simulink model "Part2"  (R2024b)
settings: Solver=VariableStepAuto  StartTime=0.0  StopTime=10  RelTol=1e-3
InitFcn:
  | % Design2
values from neighbouring files (symbols this model uses):
  Ao = F(2, 2) - L * F(1, 2)    [Design1.m]    (also in Design2.m)
  Bo = [G(2) - L * G(1), Ao * L + F(2, 1) - L * F(1, 1)]    [Design1.m]    (also in Design2.m)
  Co = [0; 1]    [Design1.m]    (also in Design2.m)
  Do = [0, 1; 0, L]    [Design1.m]    (also in Design2.m)
  K = place(F, G, DesiredPoles)    [Design1.m]    (also in Design2.m = Ktmp(2:3))
  Nr = Nu + K * Nx    [Design1.m]    (also in Design2.m)
  Ts = TsCand(i)    [Design1.m]    (also in Design2.m)
undefined symbols (not defined in the file or in its folder): DiscIntNeverNeededParam, drv, F, G, H, J, sens
libraries: simulink_extras x5
settings Model: Creator=Banaan  LastModifiedBy=Banaan

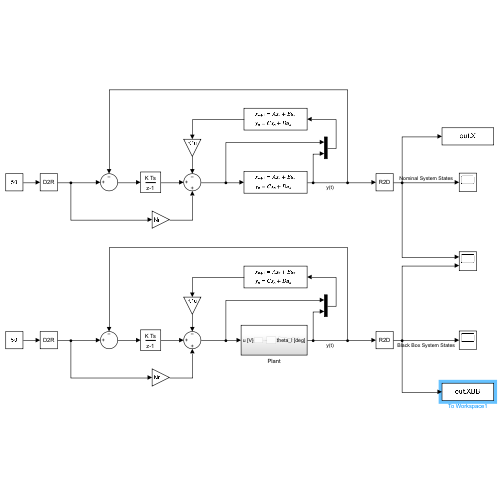
[thumbnail: Simulink's stored preview of the top-level diagram]
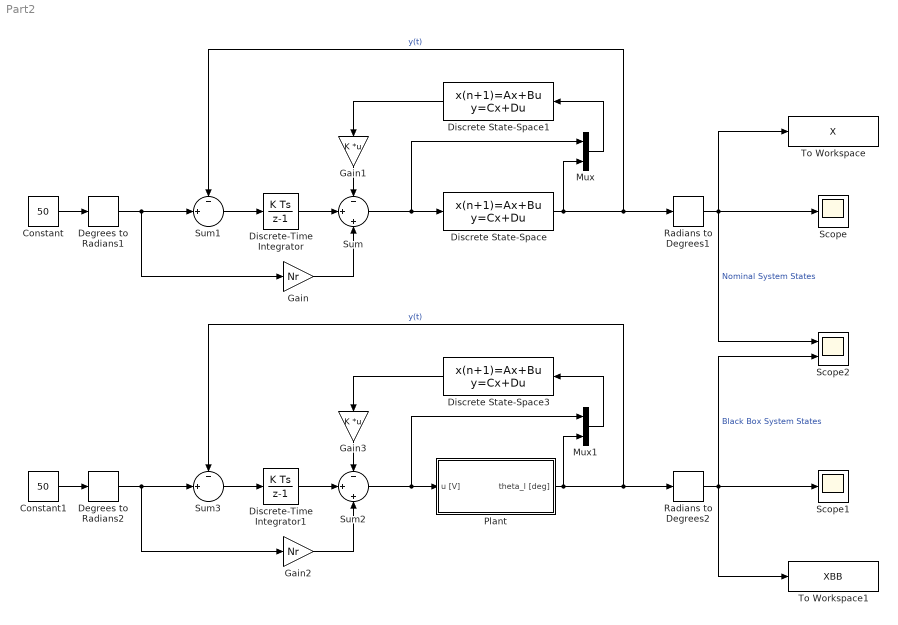
== system Part2 ==
  Constant : Constant  Value=50
  Constant1 : Constant  Value=50
  Degrees to Radians1 : simulink_extras/Transformations/Degrees to Radians
  Degrees to Radians2 : simulink_extras/Transformations/Degrees to Radians
  Discrete State-Space : DiscreteStateSpace  A=F  B=G  C=H  D=J  SampleTime=Ts
  Discrete State-Space1 : DiscreteStateSpace  A=Ao  B=Bo  C=Co  D=Do  SampleTime=Ts
  Discrete State-Space3 : DiscreteStateSpace  A=Ao  B=Bo  C=Co  D=Do  SampleTime=Ts
  Discrete-Time Integrator : DiscreteIntegrator  gainval=Ki  SampleTime=-1  ICPrevOutput=DiscIntNeverNeededParam  ICPrevScaledInput=DiscIntNeverNeededParam
  Discrete-Time Integrator1 : DiscreteIntegrator  gainval=Ki  SampleTime=-1  ICPrevOutput=DiscIntNeverNeededParam  ICPrevScaledInput=DiscIntNeverNeededParam
  Gain : Gain  Gain=Nr
  Gain1 : Gain  Gain=K  Multiplication=Matrix(K*u)
  Gain2 : Gain  Gain=Nr
  Gain3 : Gain  Gain=K  Multiplication=Matrix(K*u)
  Mux : Mux  Inputs=2
  Mux1 : Mux  Inputs=2
  Plant : Subsystem
  Radians to Degrees1 : simulink_extras/Transformations/Radians to Degrees
  Radians to Degrees2 : simulink_extras/Transformations/Radians to Degrees
  Scope : Scope
  Scope1 : Scope
  Scope2 : Scope  NumInputPorts=2
  Sum : Sum  Inputs=-|+|+
  Sum1 : Sum  Inputs=-|+||
  Sum2 : Sum  Inputs=-|+|+
  Sum3 : Sum  Inputs=-|+||
  To Workspace : ToWorkspace  VariableName=X  SaveFormat=Timeseries  SampleTime=-1
  To Workspace1 : ToWorkspace  VariableName=XBB  SaveFormat=Timeseries  SampleTime=-1
  wires:
  Constant/1 -> Degrees to Radians1/1
  Discrete State-Space/1 -> Mux/2, Radians to Degrees1/1, Sum1/1  "y(t)"
  Mux/1 -> Discrete State-Space1/1
  Sum/1 -> Mux/1, Discrete State-Space/1
  Discrete State-Space1/1 -> Gain1/1
  Gain/1 -> Sum/3
  Gain1/1 -> Sum/1
  Degrees to Radians1/1 -> Gain/1, Sum1/2
  Radians to Degrees1/1 -> To Workspace/1, Scope2/1, Scope/1  "Nominal System States"
  Discrete-Time Integrator/1 -> Sum/2
  Sum1/1 -> Discrete-Time Integrator/1
  Sum3/1 -> Discrete-Time Integrator1/1
  Discrete-Time Integrator1/1 -> Sum2/2
  Radians to Degrees2/1 -> To Workspace1/1, Scope2/2, Scope1/1  "Black Box System States"
  Degrees to Radians2/1 -> Sum3/2, Gain2/1
  Gain3/1 -> Sum2/1
  Gain2/1 -> Sum2/3
  Discrete State-Space3/1 -> Gain3/1
  Sum2/1 -> Plant/1(u [V]), Mux1/1
  Mux1/1 -> Discrete State-Space3/1
  Plant/1(theta_l [deg]) -> Sum3/1, Radians to Degrees2/1, Mux1/2  "y(t)"
  Constant1/1 -> Degrees to Radians2/1

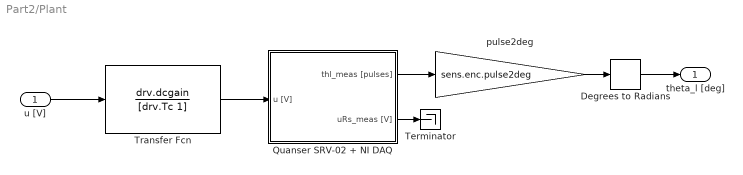
== system Part2/Plant ==
  u [V] : Inport
  Degrees to Radians : simulink_extras/Transformations/Degrees to Radians
  Quanser SRV-02 + NI DAQ : Subsystem  mask(Quanser SRV-02 (with inertial load) + NI DAQ){Ts=0.001, fricType=Coulomb + viscous}
      mask prompts: Ts "NI DAQ Sample Time:"; fricType "Friction model"
      mask help: Quanser SRV-02 (with inertial load) + NI DAQ model.
      mask init:
      | %%  Sensors data
      | 
      | %   shunt resistor
      | sens.curr.Rs = 0.5;                         %   resistance [Ohm]   
      | sens.curr.uRs_std = 0.01;                   %   voltage noise standard dev [V]                           
      | sens.curr.uRs_var = sens.curr.uRs_std^2;	%   voltage noise variance [V^2]
      | 
      | %   Hewlett-Packard HEDS-5540#A06 optical encoder
      | sens.enc.ppr = 500*4;                       %   pulses per rotation
      | sens.enc.pulse2deg = 360/sens.enc.ppr;      %   [pulses] -> [deg]
      | sens.enc.pulse2rad = 2*pi/sens.enc.ppr;     %   [pulses] -> [rad]
      | sens.enc.deg2pulse = sens.enc.ppr/360;      %   [deg] -> [pulses]
      | sens.enc.rad2pulse = sens.enc.ppr/2/pi;     %   [rad] -> [pulses]
      | 
      | 
      | %%  Data acquisition board (daq) data
      | 
      | %   NI PCI-6221 DAC data
      | daq.dac.bits = 16;                                  %   resolution (bits)
      | daq.dac.fs   = 10;                                  %   full scale 
      | daq.dac.q    = 2*daq.dac.fs/(2^daq.dac.bits-1);     %	quantization
      | 
      | %   NI PCI-6221 ADC data
      | daq.adc.bits = 16;                                  %   resolution (bits)
      | daq.adc.fs   = 10;                                  %   full scale (as set in SLDRT Analog Input block)
      | daq.adc.q    = 2*daq.adc.fs/(2^daq.adc.bits-1);     %   quantization
      mask Help:
      | Riccardo Antonello (antonello@dei.unipd.it)
      | 
      | April 24, 2020
      | 
      | Dept. of Information Engineering, University of Padova
      mask TypeOptions fricType: Coulomb + viscous | Karnopp
  Terminator : Terminator
  Transfer Fcn : TransferFcn  Numerator=drv.dcgain  Denominator=[drv.Tc 1]
  pulse2deg : Gain  Gain=sens.enc.pulse2deg
  theta_l [deg] : Outport
  wires:
  u [V]/1 -> Transfer Fcn/1
  Degrees to Radians/1 -> theta_l [deg]/1
  Quanser SRV-02 + NI DAQ/1(thl_meas [pulses]) -> pulse2deg/1
  Quanser SRV-02 + NI DAQ/2(uRs_meas [V]) -> Terminator/1
  Transfer Fcn/1 -> Quanser SRV-02 + NI DAQ/1(u [V])
  pulse2deg/1 -> Degrees to Radians/1

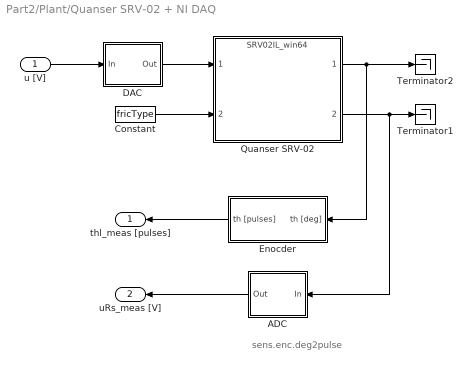
== system Part2/Plant/Quanser SRV-02 + NI DAQ ==
  note: sens.enc.deg2pulse
  u [V] : Inport
  ADC : Subsystem
  Constant : Constant  Value=fricType
  DAC : Subsystem
  Enocder : Subsystem
  Quanser SRV-02 : ModelReference  ModelNameDialog=SRV02IL_win64.slxp  ModelReferenceVersion=1.44  CopyOfModelProtected=on
  Terminator1 : Terminator
  Terminator2 : Terminator
  thl_meas [pulses] : Outport
  uRs_meas [V] : Outport  Port=2
  wires:
  Enocder/1(th [pulses]) -> thl_meas [pulses]/1
  ADC/1(Out) -> uRs_meas [V]/1
  DAC/1(Out) -> Quanser SRV-02/1
  Quanser SRV-02/2 -> ADC/1(In), Terminator1/1
  u [V]/1 -> DAC/1(In)
  Quanser SRV-02/1 -> Enocder/1(th [deg]), Terminator2/1
  Constant/1 -> Quanser SRV-02/2

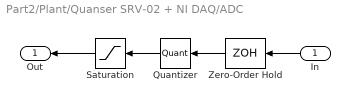
== system Part2/Plant/Quanser SRV-02 + NI DAQ/ADC ==
  In : Inport
  Quantizer : Quantizer  QuantizationInterval=daq.adc.q
  Saturation : Saturate  UpperLimit=daq.adc.fs  LowerLimit=-daq.adc.fs
  Zero-Order Hold : ZeroOrderHold  SampleTime=Ts
  Out : Outport
  wires:
  Saturation/1 -> Out/1
  In/1 -> Zero-Order Hold/1
  Quantizer/1 -> Saturation/1
  Zero-Order Hold/1 -> Quantizer/1

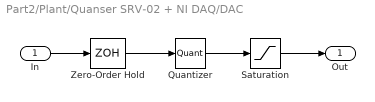
== system Part2/Plant/Quanser SRV-02 + NI DAQ/DAC ==
  In : Inport
  Quantizer : Quantizer  QuantizationInterval=daq.dac.q
  Saturation : Saturate  UpperLimit=daq.dac.fs  LowerLimit=-daq.dac.fs
  Zero-Order Hold : ZeroOrderHold  SampleTime=Ts
  Out : Outport
  wires:
  Quantizer/1 -> Saturation/1
  In/1 -> Zero-Order Hold/1
  Zero-Order Hold/1 -> Quantizer/1
  Saturation/1 -> Out/1

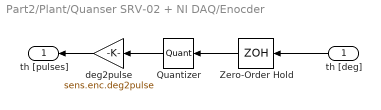
== system Part2/Plant/Quanser SRV-02 + NI DAQ/Enocder ==
  th [deg] : Inport
  Quantizer : Quantizer  QuantizationInterval=sens.enc.pulse2deg
  Zero-Order Hold : ZeroOrderHold  SampleTime=Ts
  deg2pulse : Gain  Gain=sens.enc.deg2pulse
  th [pulses] : Outport
  wires:
  Quantizer/1 -> deg2pulse/1
  th [deg]/1 -> Zero-Order Hold/1
  Zero-Order Hold/1 -> Quantizer/1
  deg2pulse/1 -> th [pulses]/1
